simulink model "T3Model"  (R2020a)
settings: Solver=ode23t  StartTime=0.0  StopTime=8800  FixedStep=0.1  RelTol=1e-3
values from neighbouring files (symbols this model uses):
  dt = T(2)-T(1)    [Consumo.m]
  Ec0 = 23.7100000000000    (= 23.71)    [Consumo.m]
  Ec10 = 0.0119000000000000    (= 0.0119)    [Consumo.m]
  Ed0 = 23.8656693114163    (= 23.8656693114)    [Consumo.m]
  Ed10 = -0.014039298384087    (= -0.0140392983841)    [Consumo.m]
  PHI0 = 374.5    [Consumo.m]
  R1 = 0.00794947264184679    (= 0.00794947264185)    [Consumo.m]
  R2 = 6.21618016293642e-05    (= 6.21618016294e-05)    [Consumo.m]
  Rc = 0.258351921779644    (= 0.25835192178)    [Consumo.m]
  Rd = 0.103662535963592    (= 0.103662535964)    [Consumo.m]
  V0 = 24    [Consumo.m]
undefined symbols (not defined in the file or in its folder): magnitude, PHI_total
libraries: fl_lib x13, nesl_utility x5
settings Model: Creator=agrc1  LastModifiedBy=Alberto
settings DebuggingCC: UnconnectedInputMsg=none  UnconnectedOutputMsg=none  UnconnectedLineMsg=none  SFMachineParentedDataDiag=error
settings ModelReferenceCC: EnableRefExpFcnMdlSchedulingChecks=off
settings RTWCC: Description=Generic Real-Time Target

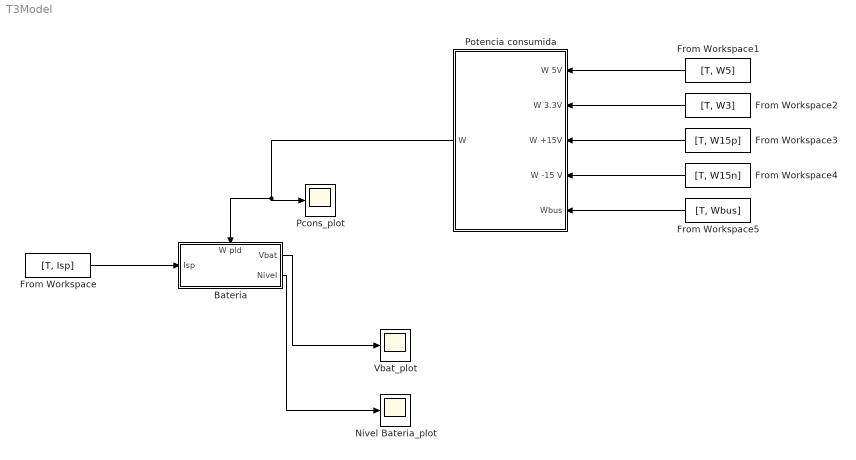
== system T3Model ==
  Bateria : Subsystem
      settings: PortSchema="{\"entries\":[{\"content\":{\"sides\":[{\"content\":{\"connectorIds\":[\"In1\"]},\"type\":\"ConnectorPlacement.EquallySpacedRectSide\",\"uuid\":\"7762626e-e995-4a2c-aa61-f41a065ba065\"},{\"content\":{\"connectorIds\":[\"Out1\",\"Out2\"],\"side\":\"RIGHT\"},\"type\":\"ConnectorPlacement.EquallySpacedRectSide\",\"uuid\":\"025bf583-2dd5-4053-bf3a-cd5569ed5285\"},{\"content\":{\"connectorIds\":[\"In2\"],\"side\":\"TOP\"},\"type\":\"ConnectorPlacement.EquallySpacedRectSide\",\"uuid\":\"d853252d-9671-4b97-85c7-0f820ff02186\"}]},\"type\":\"ConnectorPlacement.EquallySpacedConnector\",\"uuid\":\"4c05b427-12ad-4b7f-8bbf-0833b4a4ba7e\"}],\"packageUris\":[\"http://schema.mathworks.com/mf0/Connector/R2020b\"],\"version\":\"1.0\"}"
  From Workspace : FromWorkspace  VariableName=[T, Isp]  OutDataTypeStr=double  OutputAfterFinalValue=Holding final value
  From Workspace1 : FromWorkspace  VariableName=[T, W5]  OutDataTypeStr=double  OutputAfterFinalValue=Holding final value
  From Workspace2 : FromWorkspace  VariableName=[T, W3]  OutDataTypeStr=double  OutputAfterFinalValue=Holding final value
  From Workspace3 : FromWorkspace  VariableName=[T, W15p]  OutDataTypeStr=double  OutputAfterFinalValue=Holding final value
  From Workspace4 : FromWorkspace  VariableName=[T, W15n]  OutDataTypeStr=double  OutputAfterFinalValue=Holding final value
  From Workspace5 : FromWorkspace  VariableName=[T, Wbus]  OutDataTypeStr=double  OutputAfterFinalValue=Holding final value
  Nivel Bateria_plot : Scope
  Pcons_plot : Scope
  Potencia consumida : Subsystem
  Vbat_plot : Scope
  wires:
  Bateria/1(Vbat) -> Vbat_plot/1
  Bateria/2(Nivel) -> Nivel Bateria_plot/1
  From Workspace1/1 -> Potencia consumida/1(W 5V)
  From Workspace2/1 -> Potencia consumida/2(W 3.3V)
  From Workspace3/1 -> Potencia consumida/3(W +15V)
  From Workspace4/1 -> Potencia consumida/4(W -15 V)
  From Workspace5/1 -> Potencia consumida/5(Wbus)
  Potencia consumida/1(W) -> Bateria/2(W pld), Pcons_plot/1
  From Workspace/1 -> Bateria/1(Isp)

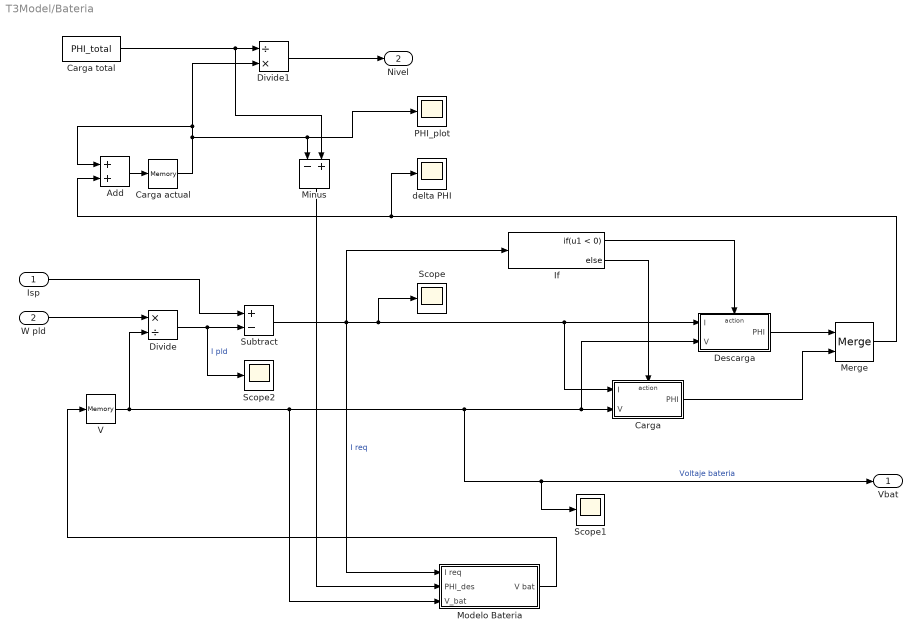
== system T3Model/Bateria ==
  Isp : Inport
  W pld : Inport  Port=2
  Add : Sum
  Carga : Subsystem  TreatAsAtomicUnit=on
  Carga actual : Memory  InitialCondition=PHI0  InheritSampleTime=on
  Carga total : Constant  Value=PHI_total
  Descarga : Subsystem  TreatAsAtomicUnit=on
  Divide : Product  Inputs=*/
  Divide1 : Product  Inputs=/*
  If : If  IfExpression=u1 < 0
  Merge : Merge
  Minus : Sum  Inputs=-+
  Modelo Bateria : Subsystem
  PHI_plot : Scope
  Scope : Scope
  Scope1 : Scope
  Scope2 : Scope
  Subtract : Sum  Inputs=+-
  V : Memory  InitialCondition=V0
  delta PHI : Scope
  Vbat : Outport
  Nivel : Outport  Port=2
  wires:
  W pld/1 -> Divide/1
  Divide/1 -> Scope2/1, Subtract/2  "I pld"
  Isp/1 -> Subtract/1
  Subtract/1 -> If/1, Modelo Bateria/1(I req), Scope/1, Carga/1(I), Descarga/1(I)  "I req"
  V/1 -> Divide/2, Scope1/1, Vbat/1, Descarga/2(V), Carga/2(V), Modelo Bateria/3(V_bat)  "Voltaje bateria"
  Descarga/1(PHI) -> Merge/1
  If/1 -> Descarga/Action
  If/2 -> Carga/Action
  Carga/1(PHI) -> Merge/2
  Carga total/1 -> Minus/2, Divide1/1
  Carga actual/1 -> PHI_plot/1, Minus/1, Add/1, Divide1/2
  Divide1/1 -> Nivel/1
  Add/1 -> Carga actual/1
  Modelo Bateria/1(V bat) -> V/1
  Merge/1 -> Add/2, delta PHI/1
  Minus/1 -> Modelo Bateria/2(PHI_des)

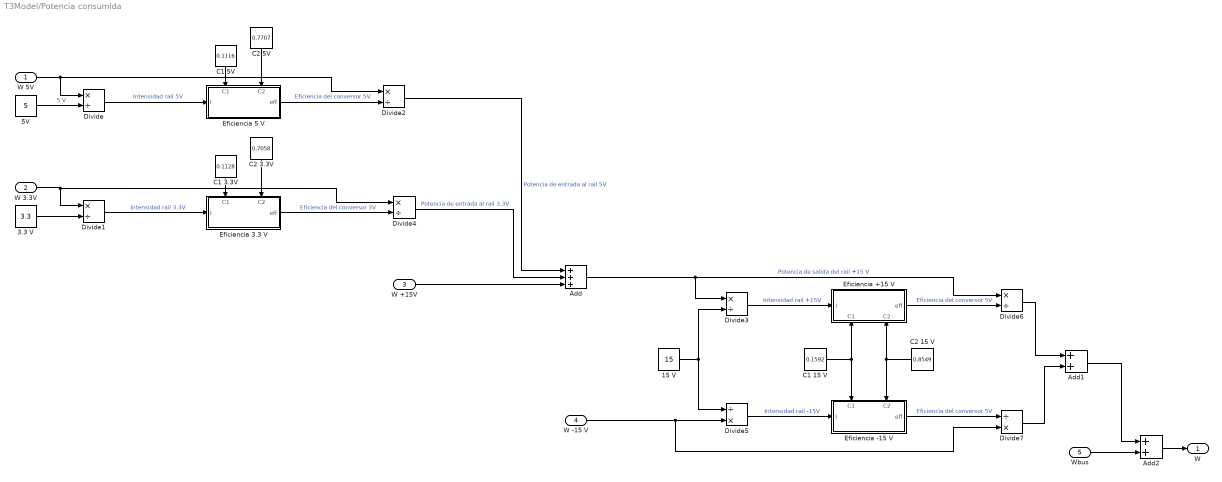
== system T3Model/Potencia consumida ==
  W 5V : Inport
  W 3.3V : Inport  Port=2
  W +15V : Inport  Port=3
  W -15 V : Inport  Port=4
  Wbus : Inport  Port=5
  15 V : Constant  Value=15
  3.3 V : Constant  Value=3.3
  5V : Constant  Value=5
  Add : Sum  Inputs=+++
  Add1 : Sum
  Add2 : Sum
  C1 15 V : Constant  Value=0.1592
  C1 3.3V : Constant  Value=0.1128
  C1 5V : Constant  Value=0.1116
  C2 15 V : Constant  Value=0.8549
  C2 3.3V : Constant  Value=0.7058
  C2 5V : Constant  Value=0.7707
  Divide{,1..4,6} (6 alike) : Product  Inputs=*/
  Divide5 : Product  Inputs=/*
  Divide7 : Product  Inputs=/*
  Eficiencia +15 V : Subsystem
      settings: PortSchema="{\"entries\":[{\"content\":{\"sides\":[{\"content\":{\"connectorIds\":[\"In1\"]},\"type\":\"ConnectorPlacement.EquallySpacedRectSide\",\"uuid\":\"b666efbc-1979-486f-b6aa-69ec31f1c5b7\"},{\"content\":{\"connectorIds\":[\"Out1\"],\"side\":\"RIGHT\"},\"type\":\"ConnectorPlacement.EquallySpacedRectSide\",\"uuid\":\"08e7998f-570d-456e-98c7-6da2ef864021\"},{\"content\":{\"connectorIds\":[],\"side\":\"TOP\"},\"type\":\"ConnectorPlacement.EquallySpacedRectSide\",\"uuid\":\"70f4c0ab-77df-46d5-b3dc-04001d3e98e7\"},{\"content\":{\"connectorIds\":[\"In2\",\"In3\"],\"side\":\"BOTTOM\"},\"type\":\"ConnectorPlacement.EquallySpacedRectSide\",\"uuid\":\"5b953f4b-6f9a-4c62-85e5-3c76240e39ce\"}]},\"type\":\"ConnectorPlacement.EquallySpacedConnector\",\"uuid\":\"91259135-ce52-4d2d-8ec3-e003adfdf9d1\"}],\"packageUris\":[\"http://schema.mathworks.com/mf0/Connector/R2020b\"],\"version\":\"1.0\"}"
  Eficiencia -15 V : Subsystem
      settings: PortSchema="{\"entries\":[{\"content\":{\"sides\":[{\"content\":{\"connectorIds\":[\"In1\"]},\"type\":\"ConnectorPlacement.EquallySpacedRectSide\",\"uuid\":\"b666efbc-1979-486f-b6aa-69ec31f1c5b7\"},{\"content\":{\"connectorIds\":[\"Out1\"],\"side\":\"RIGHT\"},\"type\":\"ConnectorPlacement.EquallySpacedRectSide\",\"uuid\":\"08e7998f-570d-456e-98c7-6da2ef864021\"},{\"content\":{\"connectorIds\":[\"In2\",\"In3\"],\"side\":\"TOP\"},\"type\":\"ConnectorPlacement.EquallySpacedRectSide\",\"uuid\":\"70f4c0ab-77df-46d5-b3dc-04001d3e98e7\"},{\"content\":{\"connectorIds\":[],\"side\":\"BOTTOM\"},\"type\":\"ConnectorPlacement.EquallySpacedRectSide\",\"uuid\":\"5b953f4b-6f9a-4c62-85e5-3c76240e39ce\"}]},\"type\":\"ConnectorPlacement.EquallySpacedConnector\",\"uuid\":\"91259135-ce52-4d2d-8ec3-e003adfdf9d1\"}],\"packageUris\":[\"http://schema.mathworks.com/mf0/Connector/R2020b\"],\"version\":\"1.0\"}"
  Eficiencia 3.3 V : Subsystem
      settings: PortSchema="{\"entries\":[{\"content\":{\"sides\":[{\"content\":{\"connectorIds\":[\"In1\"]},\"type\":\"ConnectorPlacement.EquallySpacedRectSide\",\"uuid\":\"b666efbc-1979-486f-b6aa-69ec31f1c5b7\"},{\"content\":{\"connectorIds\":[\"Out1\"],\"side\":\"RIGHT\"},\"type\":\"ConnectorPlacement.EquallySpacedRectSide\",\"uuid\":\"08e7998f-570d-456e-98c7-6da2ef864021\"},{\"content\":{\"connectorIds\":[\"In2\",\"In3\"],\"side\":\"TOP\"},\"type\":\"ConnectorPlacement.EquallySpacedRectSide\",\"uuid\":\"70f4c0ab-77df-46d5-b3dc-04001d3e98e7\"}]},\"type\":\"ConnectorPlacement.EquallySpacedConnector\",\"uuid\":\"91259135-ce52-4d2d-8ec3-e003adfdf9d1\"}],\"packageUris\":[\"http://schema.mathworks.com/mf0/Connector/R2020b\"],\"version\":\"1.0\"}"
  Eficiencia 5 V : Subsystem
      settings: PortSchema="{\"entries\":[{\"content\":{\"sides\":[{\"content\":{\"connectorIds\":[\"In1\"]},\"type\":\"ConnectorPlacement.EquallySpacedRectSide\",\"uuid\":\"b666efbc-1979-486f-b6aa-69ec31f1c5b7\"},{\"content\":{\"connectorIds\":[\"Out1\"],\"side\":\"RIGHT\"},\"type\":\"ConnectorPlacement.EquallySpacedRectSide\",\"uuid\":\"08e7998f-570d-456e-98c7-6da2ef864021\"},{\"content\":{\"connectorIds\":[\"In2\",\"In3\"],\"side\":\"TOP\"},\"type\":\"ConnectorPlacement.EquallySpacedRectSide\",\"uuid\":\"70f4c0ab-77df-46d5-b3dc-04001d3e98e7\"}]},\"type\":\"ConnectorPlacement.EquallySpacedConnector\",\"uuid\":\"91259135-ce52-4d2d-8ec3-e003adfdf9d1\"}],\"packageUris\":[\"http://schema.mathworks.com/mf0/Connector/R2020b\"],\"version\":\"1.0\"}"
  W : Outport
  wires:
  5V/1 -> Divide/2  "5 V"
  C1 5V/1 -> Eficiencia 5 V/2(C1)
  C2 5V/1 -> Eficiencia 5 V/3(C2)
  W 5V/1 -> Divide2/1, Divide/1
  Divide/1 -> Eficiencia 5 V/1(I)  "Intensidad rail 5V"
  C1 3.3V/1 -> Eficiencia 3.3 V/2(C1)
  W 3.3V/1 -> Divide4/1, Divide1/1
  Divide1/1 -> Eficiencia 3.3 V/1(I)  "Intensidad rail 3.3V"
  C2 3.3V/1 -> Eficiencia 3.3 V/3(C2)
  3.3 V/1 -> Divide1/2
  Eficiencia 5 V/1(eff) -> Divide2/2  "Eficiencia del conversor 5V"
  Divide2/1 -> Add/1  "Potencia de entrada al rail 5V"
  Eficiencia 3.3 V/1(eff) -> Divide4/2  "Eficiencia del conversor 3V"
  Divide4/1 -> Add/2  "Potencia de entrada al rail 3.3V"
  W +15V/1 -> Add/3
  Add/1 -> Divide6/1, Divide3/1  "Potencia de salida del rail +15 V"
  Divide3/1 -> Eficiencia +15 V/1(I)  "Intensidad rail +15V"
  C2 15 V/1 -> Eficiencia +15 V/3(C2), Eficiencia -15 V/3(C2)
  C1 15 V/1 -> Eficiencia +15 V/2(C1), Eficiencia -15 V/2(C1)
  W -15 V/1 -> Divide7/2, Divide5/2
  15 V/1 -> Divide3/2, Divide5/1
  Divide5/1 -> Eficiencia -15 V/1(I)  "Intensidad rail -15V"
  Eficiencia +15 V/1(eff) -> Divide6/2  "Eficiencia del conversor 5V"
  Divide6/1 -> Add1/1
  Eficiencia -15 V/1(eff) -> Divide7/1  "Eficiencia del conversor 5V"
  Divide7/1 -> Add1/2
  Add1/1 -> Add2/1
  Add2/1 -> W/1
  Wbus/1 -> Add2/2

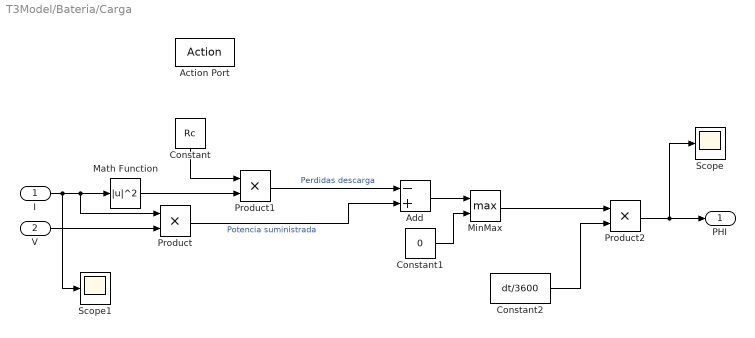
== system T3Model/Bateria/Carga ==
  I : Inport
  V : Inport  Port=2
  Action Port : ActionPort  ActionPortLabel=else
  Add : Sum  Inputs=-+
  Constant : Constant  Value=Rc
  Constant1 : Constant  Value=0
  Constant2 : Constant  Value=dt/3600
  Math Function : Math  Operator=magnitude^2  SaturateOnIntegerOverflow=on
  MinMax : MinMax  Function=max  Inputs=2
  Product : Product
  Product1 : Product
  Product2 : Product
  Scope : Scope
  Scope1 : Scope
  PHI : Outport
  wires:
  I/1 -> Scope1/1, Product/1, Math Function/1
  Product1/1 -> Add/1  "Perdidas descarga"
  Math Function/1 -> Product1/2
  Constant/1 -> Product1/1
  V/1 -> Product/2
  Product/1 -> Add/2  "Potencia suministrada"
  Add/1 -> MinMax/1
  Constant1/1 -> MinMax/2
  MinMax/1 -> Product2/1
  Product2/1 -> Scope/1, PHI/1
  Constant2/1 -> Product2/2

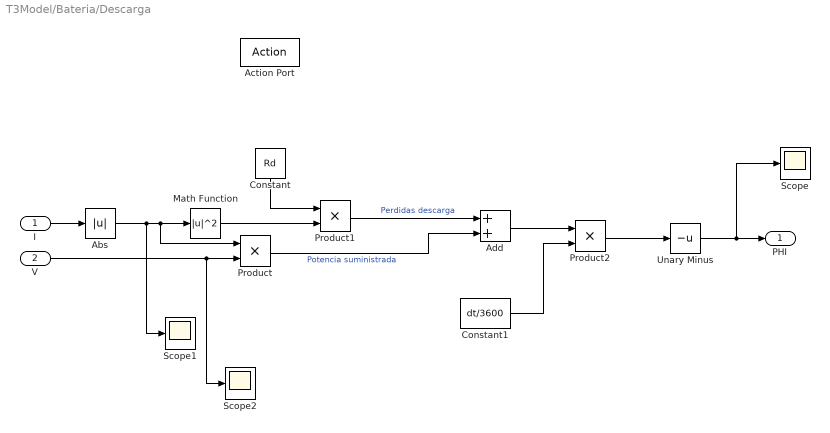
== system T3Model/Bateria/Descarga ==
  I : Inport
  V : Inport  Port=2
  Action Port : ActionPort  ActionPortLabel=if(u1 < 0)
  Abs : Abs
  Add : Sum
  Constant : Constant  Value=Rd
  Constant1 : Constant  Value=dt/3600
  Math Function : Math  Operator=magnitude^2  SaturateOnIntegerOverflow=on
  Product : Product
  Product1 : Product
  Product2 : Product
  Scope : Scope
  Scope1 : Scope
  Scope2 : Scope
  Unary Minus : UnaryMinus
  PHI : Outport
  wires:
  Math Function/1 -> Product1/2
  Product/1 -> Add/2  "Potencia suministrada"
  Constant/1 -> Product1/1
  Product1/1 -> Add/1  "Perdidas descarga"
  I/1 -> Abs/1
  V/1 -> Scope2/1, Product/2
  Add/1 -> Product2/1
  Product2/1 -> Unary Minus/1
  Constant1/1 -> Product2/2
  Abs/1 -> Scope1/1, Product/1, Math Function/1
  Unary Minus/1 -> Scope/1, PHI/1

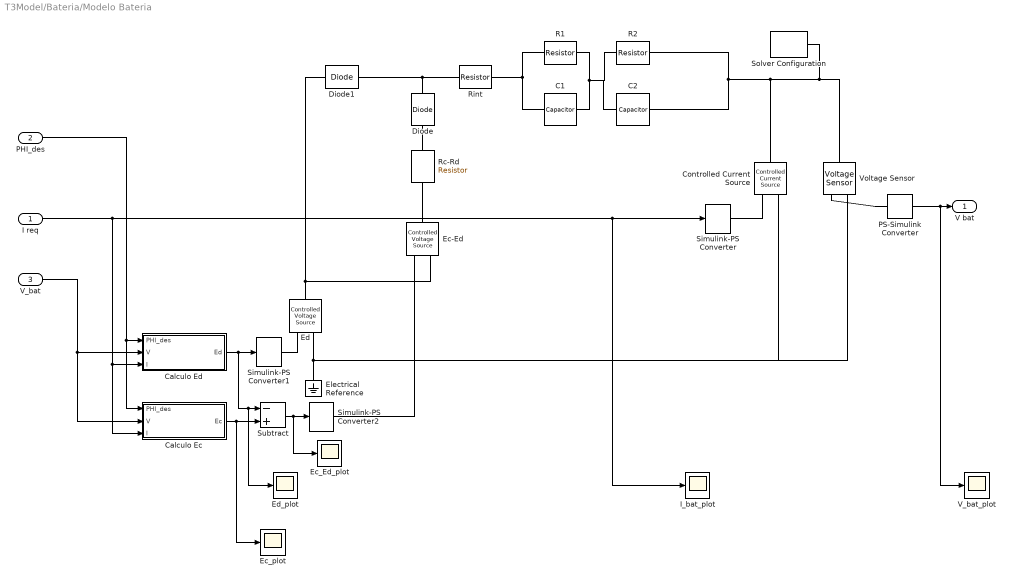
== system T3Model/Bateria/Modelo Bateria ==
  I req : Inport
  PHI_des : Inport  Port=2
  V_bat : Inport  Port=3
  C1 : fl_lib/Electrical/Electrical Elements/Capacitor  c=C1 F  r=1e-12 Ohm  g=1e-12 1/Ohm  i_specify=off  i_priority=High  i=0 A  i_nominal_specify=off  i_nominal_unit=A  i_nominal_value=1  v_specify=off  v_priority=High  v=0 V  v_nominal_specify=off  v_nominal_unit=V  v_nominal_value=1  vc_specify=off  vc_priority=High  vc=0 V  vc_nominal_specify=off  vc_nominal_unit=V  vc_nominal_value=1
  C2 : fl_lib/Electrical/Electrical Elements/Capacitor  c=C2 F  r=1e-12 Ohm  g=1e-12 1/Ohm  i_specify=off  i_priority=High  i=0 A  i_nominal_specify=off  i_nominal_unit=A  i_nominal_value=1  v_specify=off  v_priority=High  v=0 V  v_nominal_specify=off  v_nominal_unit=V  v_nominal_value=1  vc_specify=off  vc_priority=High  vc=0 V  vc_nominal_specify=off  vc_nominal_unit=V  vc_nominal_value=1
  Calculo Ec : Subsystem
  Calculo Ed : Subsystem
  Controlled Current Source : fl_lib/Electrical/Electrical Sources/Controlled Current Source
  Diode : fl_lib/Electrical/Electrical Elements/Diode  Vf=1e-12 V  Ron=1e-12 Ohm  Goff=1e-12 1/Ohm  i_specify=off  i_priority=None  i=0 A  i_nominal_specify=off  i_nominal_unit=A  i_nominal_value=1  v_specify=off  v_priority=None  v=0 V  v_nominal_specify=off  v_nominal_unit=V  v_nominal_value=1
  Diode1 : fl_lib/Electrical/Electrical Elements/Diode  Vf=1e-12 V  Ron=1e-12 Ohm  Goff=1e-12 1/Ohm  i_specify=off  i_priority=None  i=0 A  i_nominal_specify=off  i_nominal_unit=A  i_nominal_value=1  v_specify=off  v_priority=None  v=0 V  v_nominal_specify=off  v_nominal_unit=V  v_nominal_value=1
  Ec-Ed : fl_lib/Electrical/Electrical Sources/Controlled Voltage Source
  Ec_Ed_plot : Scope
  Ec_plot : Scope
  Ed : fl_lib/Electrical/Electrical Sources/Controlled Voltage Source
  Ed_plot : Scope
  Electrical Reference : fl_lib/Electrical/Electrical Elements/Electrical Reference
  I_bat_plot : Scope
  PS-Simulink Converter : nesl_utility/PS-Simulink Converter  PhysicalDomain=network_engine_domain  SubClassName=ps_output  LeftPortType=input  RightPortType=output  PseudoPeriodic=off  Frequencies=[]  Unit=V  AffineConversion=off
  R1 : fl_lib/Electrical/Electrical Elements/Resistor  R=R1 Ohm  i_specify=off  i_priority=High  i=0 A  i_nominal_specify=off  i_nominal_unit=A  i_nominal_value=1  v_specify=off  v_priority=High  v=0 V  v_nominal_specify=off  v_nominal_unit=V  v_nominal_value=1
  R2 : fl_lib/Electrical/Electrical Elements/Resistor  R=R2 Ohm  i_specify=off  i_priority=High  i=0 A  i_nominal_specify=off  i_nominal_unit=A  i_nominal_value=1  v_specify=off  v_priority=High  v=0 V  v_nominal_specify=off  v_nominal_unit=V  v_nominal_value=1
  Rc-Rd : fl_lib/Electrical/Electrical Elements/Resistor  R=Rc-Rd Ohm  i_specify=off  i_priority=High  i=0 A  i_nominal_specify=off  i_nominal_unit=A  i_nominal_value=1  v_specify=off  v_priority=High  v=0 V  v_nominal_specify=off  v_nominal_unit=V  v_nominal_value=1
  Rint : fl_lib/Electrical/Electrical Elements/Resistor  R=Rd-R1-R2 Ohm  i_specify=off  i_priority=High  i=0 A  i_nominal_specify=off  i_nominal_unit=A  i_nominal_value=1  v_specify=off  v_priority=High  v=0 V  v_nominal_specify=off  v_nominal_unit=V  v_nominal_value=1
  Simulink-PS Converter : nesl_utility/Simulink-PS Converter  PhysicalDomain=network_engine_domain  SubClassName=ps_input  LeftPortType=input  RightPortType=output  PseudoPeriodic=off  Frequencies=[]  NoiseDistribution=none  NoiseParameters=[]  Unit=A  AffineConversion=off  FilteringAndDerivatives=zero  SimscapeFilterOrder=1  InputFilterTimeConstant=0.001  UdotUserProvided=1
  Simulink-PS Converter1 : nesl_utility/Simulink-PS Converter  PhysicalDomain=network_engine_domain  SubClassName=ps_input  LeftPortType=input  RightPortType=output  PseudoPeriodic=off  Frequencies=[]  NoiseDistribution=none  NoiseParameters=[]  Unit=V  AffineConversion=off  FilteringAndDerivatives=zero  SimscapeFilterOrder=1  InputFilterTimeConstant=0.001  UdotUserProvided=1
  Simulink-PS Converter2 : nesl_utility/Simulink-PS Converter  PhysicalDomain=network_engine_domain  SubClassName=ps_input  LeftPortType=input  RightPortType=output  PseudoPeriodic=off  Frequencies=[]  NoiseDistribution=none  NoiseParameters=[]  Unit=V  AffineConversion=off  FilteringAndDerivatives=zero  SimscapeFilterOrder=1  InputFilterTimeConstant=0.001  UdotUserProvided=1
  Solver Configuration : nesl_utility/Solver Configuration  PhysicalDomain=network_engine_domain  SubClassName=solver  LeftPortType=input  RightPortType=generic  Tones=[]  Harmonics=[]  SimulateNoise=off  Profile=off  UseLocalSampling=off  EnableSwitchedLinearOptims=on  FrequencyDomain=off  UseCCode=off  RelTol=0.001  AbsTol=1e-06  MinStep=1e-09  ToWorkspace=off  RevertToSquareIcSolve=off  NumHomotopyIterations=100  PhasorMode=off  PhasorModeNumHarmonics=1  DoDC=off  ResidualTolerance=1e-9  UseLocalSolver=off  LocalSolverChoice=NE_BACKWARD_EULER_ADVANCER  LocalSolverSampleTime=0.001  DoFixedCost=off  MaxNonlinIter=3  MaxModeIter=2  LinearAlgebra=Sparse  EquationFormulation=NE_TIME_EF  DelaysMemoryBudget=1024  AutomaticFiltering=on  FilteringTimeConstant=0.001  PartitionStorageMethod=AS_NEEDED  PartitionMemoryBudget=1024  PartitionMethod=FAST
  Subtract : Sum  Inputs=-+
  V_bat_plot : Scope
  Voltage Sensor : fl_lib/Electrical/Electrical Sensors/Voltage Sensor
  V bat : Outport
  wires:
  Calculo Ec/1(Ec) -> Ec_plot/1, Subtract/2
  Calculo Ed/1(Ed) -> Ed_plot/1, Subtract/1, Simulink-PS Converter1/1
  Subtract/1 -> Ec_Ed_plot/1, Simulink-PS Converter2/1
  I req/1 -> Calculo Ec/3(I), Calculo Ed/3(I), I_bat_plot/1, Simulink-PS Converter/1
  PS-Simulink Converter/1 -> V_bat_plot/1, V bat/1
  PHI_des/1 -> Calculo Ec/1(PHI_des), Calculo Ed/1(PHI_des)
  V_bat/1 -> Calculo Ec/2(V), Calculo Ed/2(V)
  connections:
  R1/LConn1 -- C1/RConn1 -- Rint/LConn1
  Diode/LConn1 -- Rint/RConn1 -- Diode1/RConn1
  R1/RConn1 -- R2/LConn1 -- C2/RConn1 -- C1/LConn1
  Ec-Ed/RConn2 -- Ed/LConn1 -- Diode1/LConn1
  C2/LConn1 -- Solver Configuration/RConn1 -- Voltage Sensor/LConn1 -- Controlled Current Source/LConn1 -- R2/RConn1
  Ec-Ed/LConn1 -- Rc-Rd/LConn1
  Diode/RConn1 -- Rc-Rd/RConn1
  Simulink-PS Converter1/RConn1 -- Ed/RConn1
  Simulink-PS Converter2/RConn1 -- Ec-Ed/RConn1
  Electrical Reference/LConn1 -- Controlled Current Source/RConn2 -- Voltage Sensor/RConn2 -- Ed/RConn2
  Simulink-PS Converter/RConn1 -- Controlled Current Source/RConn1
  PS-Simulink Converter/LConn1 -- Voltage Sensor/RConn1

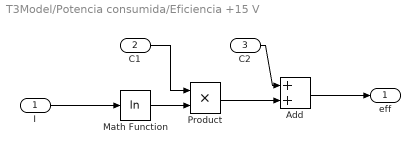
== system T3Model/Potencia consumida/Eficiencia +15 V ==
  I : Inport
  C1 : Inport  Port=2
  C2 : Inport  Port=3
  Add : Sum
  Math Function : Math  Operator=log  SaturateOnIntegerOverflow=on
  Product : Product
  eff : Outport
  wires:
  I/1 -> Math Function/1
  Math Function/1 -> Product/2
  C1/1 -> Product/1
  Product/1 -> Add/2
  Add/1 -> eff/1
  C2/1 -> Add/1

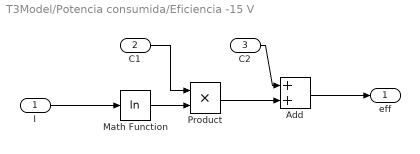
== system T3Model/Potencia consumida/Eficiencia -15 V ==
  I : Inport
  C1 : Inport  Port=2
  C2 : Inport  Port=3
  Add : Sum
  Math Function : Math  Operator=log  SaturateOnIntegerOverflow=on
  Product : Product
  eff : Outport
  wires:
  I/1 -> Math Function/1
  Math Function/1 -> Product/2
  C1/1 -> Product/1
  Product/1 -> Add/2
  Add/1 -> eff/1
  C2/1 -> Add/1

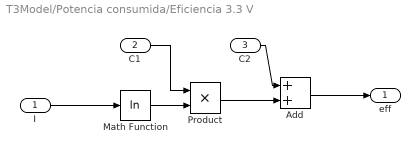
== system T3Model/Potencia consumida/Eficiencia 3.3 V ==
  I : Inport
  C1 : Inport  Port=2
  C2 : Inport  Port=3
  Add : Sum
  Math Function : Math  Operator=log  SaturateOnIntegerOverflow=on
  Product : Product
  eff : Outport
  wires:
  I/1 -> Math Function/1
  Math Function/1 -> Product/2
  C1/1 -> Product/1
  Product/1 -> Add/2
  Add/1 -> eff/1
  C2/1 -> Add/1

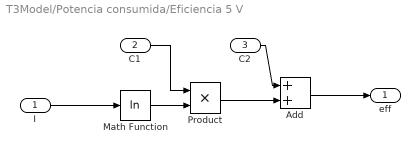
== system T3Model/Potencia consumida/Eficiencia 5 V ==
  I : Inport
  C1 : Inport  Port=2
  C2 : Inport  Port=3
  Add : Sum
  Math Function : Math  Operator=log  SaturateOnIntegerOverflow=on
  Product : Product
  eff : Outport
  wires:
  I/1 -> Math Function/1
  Math Function/1 -> Product/2
  C1/1 -> Product/1
  Product/1 -> Add/2
  Add/1 -> eff/1
  C2/1 -> Add/1

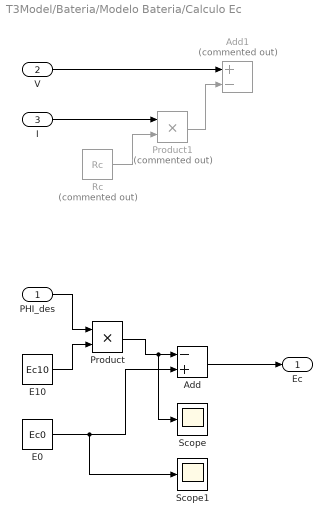
== system T3Model/Bateria/Modelo Bateria/Calculo Ec ==
  PHI_des : Inport
  V : Inport  Port=2
  I : Inport  Port=3
  Add : Sum  Inputs=-+
  Add1 : Sum  Commented=on  Inputs=+-
  E0 : Constant  Value=Ec0
  E10 : Constant  Value=Ec10
  Product : Product
  Product1 : Product  Commented=on
  Rc : Constant  Commented=on  Value=Rc
  Scope : Scope
  Scope1 : Scope
  Ec : Outport
  wires:
  Product/1 -> Scope/1, Add/1
  E10/1 -> Product/2
  E0/1 -> Scope1/1, Add/2
  I/1 -> Product1/1
  Rc/1 -> Product1/2
  V/1 -> Add1/1
  Product1/1 -> Add1/2
  PHI_des/1 -> Product/1
  Add/1 -> Ec/1

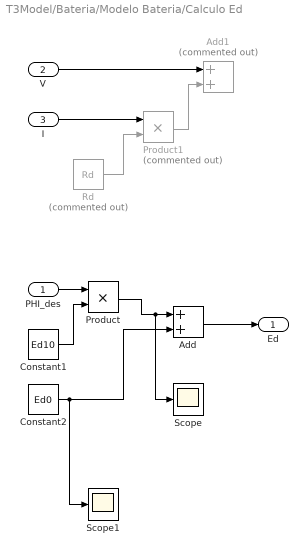
== system T3Model/Bateria/Modelo Bateria/Calculo Ed ==
  PHI_des : Inport
  V : Inport  Port=2
  I : Inport  Port=3
  Add : Sum
  Add1 : Sum  Commented=on
  Constant1 : Constant  Value=Ed10
  Constant2 : Constant  Value=Ed0
  Product : Product
  Product1 : Product  Commented=on
  Rd : Constant  Commented=on  Value=Rd
  Scope : Scope
  Scope1 : Scope
  Ed : Outport
  wires:
  Product/1 -> Scope/1, Add/1
  Constant1/1 -> Product/2
  Constant2/1 -> Scope1/1, Add/2
  I/1 -> Product1/1
  Rd/1 -> Product1/2
  V/1 -> Add1/1
  Product1/1 -> Add1/2
  PHI_des/1 -> Product/1
  Add/1 -> Ed/1
